simulink model "Simulink_Observation_5"  (R2020b)
settings: Solver=VariableStepAuto  StartTime=0.0  StopTime=0  RelTol=1e-3
settings Model: Creator=Mohit Akhouri  LastModifiedBy=Mohit Akhouri

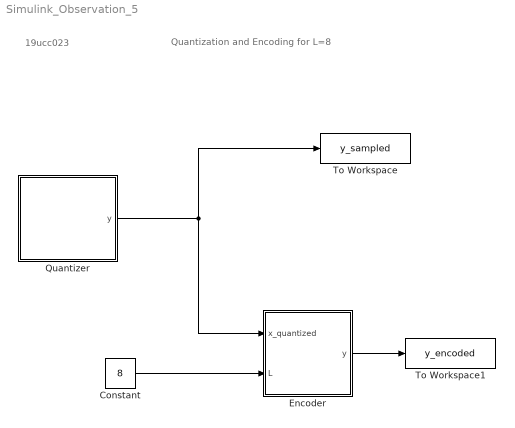
== system Simulink_Observation_5 ==
  note: Quantization and Encoding for L=8
  note: 19ucc023
  Constant : Constant  Value=8
  Encoder : MATLAB Function  TreatAsAtomicUnit=on
  Quantizer : MATLAB Function  TreatAsAtomicUnit=on
  To Workspace : ToWorkspace  VariableName=y_sampled  SaveFormat=Timeseries  SampleTime=-1
  To Workspace1 : ToWorkspace  VariableName=y_encoded  SaveFormat=Timeseries  SampleTime=-1
  wires:
  Quantizer/1(y) -> Encoder/1(x_quantized), To Workspace/1
  Constant/1 -> Encoder/2(L)
  Encoder/1(y) -> To Workspace1/1

== matlab function Simulink_Observation_5/Quantizer ==
  data: y output
function y  = fcn()

n_cycles = 5; % defining number of cycles
f = 3000; % defining message signal frequency
fs_sampled = 8000; % defining Sampling frequency
A = 1; % defining Amplitude
L = 8; % defining number of levels for the quantizer

n_sampled = 0:1:floor(n_cycles*(fs_sampled/f))-1; % defining the range of "n"
x_sampled = A*cos(2*pi*f*n_sampled*(1/fs_sampled)); % defining the sampled signal

max_value = max(x_sampled); % maximum value of sampled signal
min_value = min(x_sampled); % minimum value of sampled signal
delta = (max_value - min_value)/L; % Step size ( delta ) calculation

len = length(x_sampled); % defining length of sampled signal

y = zeros(1,len);
for ind = 1:len
    i = round((x_sampled(ind)-min_value)/delta); % calculating value of i
    y(ind) = min_value + i*delta; % calculating and storing quantized value of ith sample of x_sampled
end

== matlab function Simulink_Observation_5/Encoder ==
  data: x_quantized input; y output; L input
function y = fcn(x_quantized,L)

max_value = max(x_quantized); % maximum value of sampled signal
min_value = min(x_quantized); % minimum value of sampled signal
delta = (max_value - min_value)/(L-1); % Step size ( delta ) calculation

len = length(x_quantized); % calculating length of x_quantized
y = zeros(1,len);

for ind=1:len
    i = (x_quantized(ind)-min_value)/delta; % calculating the decimal value for encoding
    str = dec2bin(i,3); % converting decimal number i to binary number
    y(ind) = bin2dec(str);
end
